simulink model "Project_tank_in_series_MPC_control"  (R2019b)
settings: Solver=VariableStepAuto  StartTime=0.0  StopTime=t5  RelTol=1e-3
values from neighbouring files (symbols this model uses):
  C = 2.4    [heated_tank_in_series.m]
  q1 = 50    [heated_tank_in_series.m]
  q2 = 50    [heated_tank_in_series.m]
  q2_1 = -60    [heated_tank_in_series.m]
  q2_2 = +60    (= 60)    [heated_tank_in_series.m]
  q2_3 = +60    (= 60)    [heated_tank_in_series.m]
  q2_4 = -60    [heated_tank_in_series.m]
  q_out = q1+q2    (= 100)    [heated_tank_in_series.m]
  rho = 1000    [heated_tank_in_series.m]
  t1 = 30    [heated_tank_in_series.m]
  T1_1 = -0.5    [heated_tank_in_series.m]
  T1_2 = +0.5    (= 0.5)    [heated_tank_in_series.m]
  T1_3 = +0.5    (= 0.5)    [heated_tank_in_series.m]
  T1_4 = -0.5    [heated_tank_in_series.m]
  T2 = 6    [heated_tank_in_series.m]
  t2 = 60    [heated_tank_in_series.m]
  t3 = 90    [heated_tank_in_series.m]
  T3_0 = (((q1*T1_0/V) + (q2*T2/V)))*(V/q_out)    (= 5)    [heated_tank_in_series.m]
  t4 = 120    [heated_tank_in_series.m]
  T4_0 = double(solve(T4_eq, T4_0))    [heated_tank_in_series.m]
  Th_1 = -5    [heated_tank_in_series.m]
  Th_2 = +5    (= 5)    [heated_tank_in_series.m]
  Th_3 = +5    (= 5)    [heated_tank_in_series.m]
  Th_4 = -5    [heated_tank_in_series.m]
  UA = 5*10^4    (= 50000)    [heated_tank_in_series.m]
  V = 100    [heated_tank_in_series.m]
libraries: mpclib x1
settings Model: Creator=oasys  LastModifiedBy=oasys

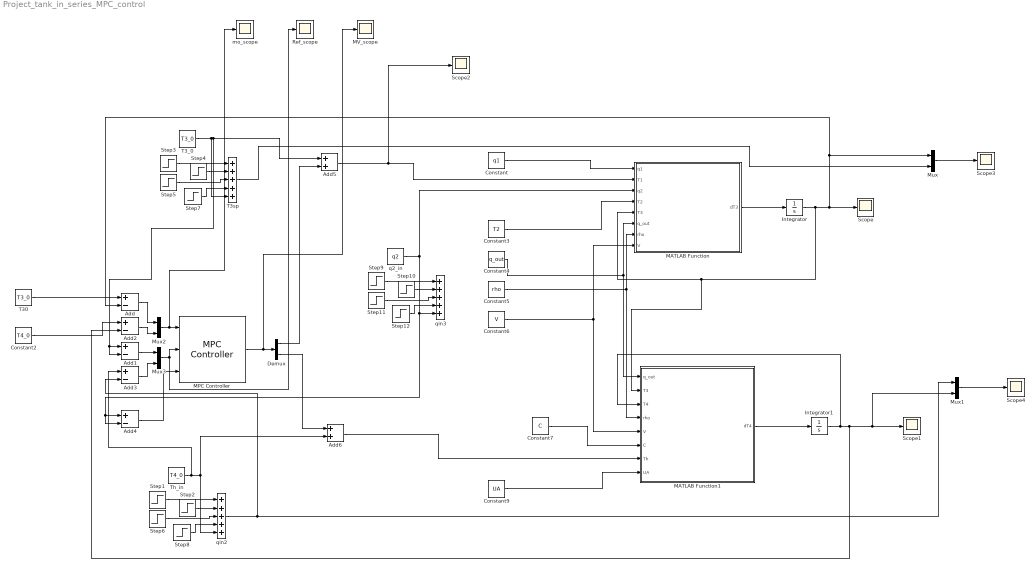
== system Project_tank_in_series_MPC_control ==
  Add{,1..4} (5 alike) : Sum  Inputs=+-
  Add5 : Sum
  Add6 : Sum
  Constant : Constant  Value=q1
  Constant2 : Constant  Value=T4_0
  Constant3 : Constant  Value=T2
  Constant4 : Constant  Value=q_out
  Constant5 : Constant  Value=rho
  Constant6 : Constant  Value=V
  Constant7 : Constant  Value=C
  Constant9 : Constant  Value=UA
  Demux : Demux  Outputs=2
  Integrator : Integrator  InitialCondition=T3_0
  Integrator1 : Integrator  InitialCondition=T4_0
  MATLAB Function : MATLAB Function  TreatAsAtomicUnit=on
  MATLAB Function1 : MATLAB Function  TreatAsAtomicUnit=on
  MPC Controller : mpclib/MPC Controller  SCDEnableBlockLinearizationSpecification=on  mpcobj=mpcB  x0=xmpcB  is_multiple=0  enable_value=0  return_u0=off  updateMPCinCallerWorkspace=on  md_inport=on  mv_inport=off  uref_inport=off  return_cost=off  return_mvseq=off  return_qpstatus=off  return_xseq=off  return_state=off  return_ovseq=off  state_inport=off  umin_inport=off  umax_inport=off  ymin_inport=off  ymax_inport=off  cc_inport=off  ywt_inport=off  uwt_inport=off  duwt_inport=off  rhoeps_inport=off  pm_inport=off  MaximumP=10  HorizonChoice=FixedHorizon  n_ts=0.5  n_p=30  n_mv=2  n_md=1  n_ud=0  n_mo=2  n_uo=0  BlockDataType=double  SampleTimeInherited=off  switch_inport=off
  MV_scope : Scope
  Mux{,1..3} (4 alike) : Mux  Inputs=2
  Ref_scope : Scope
  Scope{,1..4} (5 alike) : Scope
  Step1 : Step  Time=t1  After=Th_1  SampleTime=0
  Step10 : Step  Time=t2  After=q2_2  SampleTime=0
  Step11 : Step  Time=t3  After=q2_3  SampleTime=0
  Step12 : Step  Time=t4  After=q2_4  SampleTime=0
  Step2 : Step  Time=t2  After=Th_2  SampleTime=0
  Step3 : Step  Time=t1  After=T1_1  SampleTime=0
  Step4 : Step  Time=t2  After=T1_2  SampleTime=0
  Step5 : Step  Time=t3  After=T1_3  SampleTime=0
  Step6 : Step  Time=t3  After=Th_3  SampleTime=0
  Step7 : Step  Time=t4  After=T1_4  SampleTime=0
  Step8 : Step  Time=t4  After=Th_4  SampleTime=0
  Step9 : Step  Time=t1  After=q2_1  SampleTime=0
  "T30 " : Constant  Value=T3_0
  T3_0 : Constant  Value=T3_0
  T3sp : Sum  Inputs=+++++
  Th_in : Constant  Value=T4_0
  mo_scope : Scope
  q2_in : Constant  Value=q2
  qin2 : Sum  Inputs=+++++
  qin3 : Sum  Inputs=+++++
  wires:
  Mux/1 -> Scope3/1
  Constant6/1 -> MATLAB Function/8(V), MATLAB Function1/5(V)
  Integrator1/1 -> Add2/2, Mux1/2, Scope1/1, MATLAB Function1/3(T4)
  MATLAB Function1/1(dT4) -> Integrator1/1
  Constant7/1 -> MATLAB Function1/6(C)
  Constant5/1 -> MATLAB Function1/4(rho), MATLAB Function/7(rho)
  Constant/1 -> MATLAB Function/1(q1)
  Constant4/1 -> MATLAB Function/6(q_out), MATLAB Function1/1(q_out)
  Step11/1 -> qin3/3
  T3_0/1 -> Add1/1, Add1/2, Add5/1, T3sp/5
  Integrator/1 -> Add/2, Mux/1, Scope/1, MATLAB Function/5(T3), MATLAB Function1/2(T3)
  Constant3/1 -> MATLAB Function/4(T2)
  Mux1/1 -> Scope4/1
  Step5/1 -> T3sp/3
  Step12/1 -> qin3/4
  Step2/1 -> qin2/2
  Step1/1 -> qin2/1
  Step8/1 -> qin2/4
  Step4/1 -> T3sp/2
  q2_in/1 -> Add4/2, Add4/1, qin3/5, MATLAB Function/3(q2)
  Constant9/1 -> MATLAB Function1/8(UA)
  Th_in/1 -> Add3/1, Add6/2, qin2/5
  Step7/1 -> T3sp/4
  MATLAB Function/1(dT3) -> Integrator/1
  Step9/1 -> qin3/1
  Step3/1 -> T3sp/1
  Step10/1 -> qin3/2
  Step6/1 -> qin2/3
  MPC Controller/1 -> MV_scope/1, Demux/1
  Mux2/1 -> mo_scope/1, MPC Controller/1
  Add/1 -> Mux2/1
  Add2/1 -> Mux2/2
  Mux3/1 -> MPC Controller/2, Ref_scope/1
  Add1/1 -> Mux3/1
  Add3/1 -> Mux3/2
  Add4/1 -> MPC Controller/3
  Demux/1 -> Add5/2
  Add5/1 -> Scope2/1, MATLAB Function/2(T1)
  Demux/2 -> Add6/1
  Add6/1 -> MATLAB Function1/7(Th)
  "T30 "/1 -> Add/1
  Constant2/1 -> Add2/1
  qin2/1 -> Add3/2, Mux1/1
  T3sp/1 -> Mux/2

== matlab function Project_tank_in_series_MPC_control/MATLAB Function1 ==
  data: q_out input; dT4 output; T3 input; T4 input; rho input; V input; C input; Th input; UA input
function dT4 = T4(q_out,T3,T4,rho,V,C,Th,UA)
Q = UA*(Th-T4);
dT4 =(q_out*rho*C*(T3 - T4) + Q)/(rho*V*C);

== matlab function Project_tank_in_series_MPC_control/MATLAB Function ==
  data: q1 input; dT3 output; T1 input; q2 input; T2 input; T3 input; q_out input; rho input; V input
function dT3 = T3(q1,T1,q2,T2,T3,q_out,rho,V)

dT3 = (T1*q1*rho + T2*q2*rho - T3*q_out*rho)/(rho*V);
